simulink model "nonlinear_ss_control_with_reference"  (R2019b)
settings: Solver=ode45  StartTime=0.0  StopTime=700.0  MaxStep=0.001  RelTol=1e-8
settings Model: Creator=Hector  LastModifiedBy=Hector

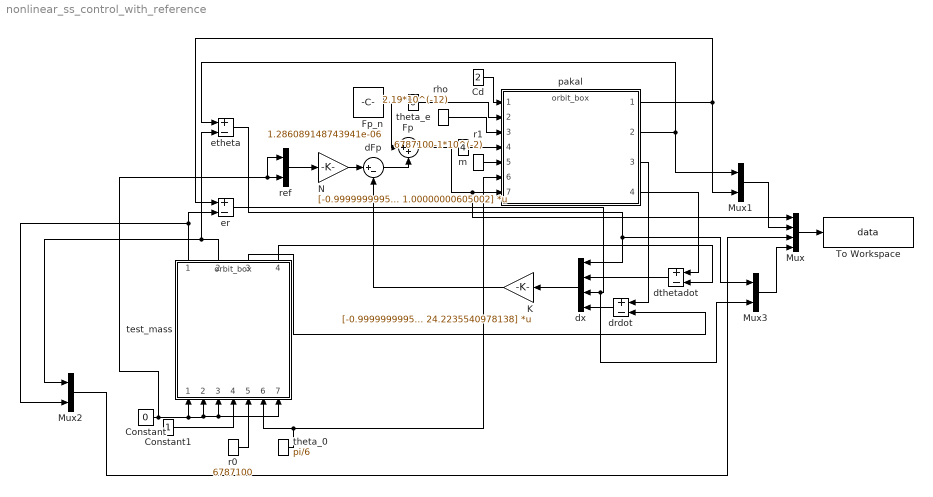
== system nonlinear_ss_control_with_reference ==
  Cd : Constant  Value=2
  Constant : Constant  Value=0
  Constant1 : Constant
  Fp : Sum  Inputs=|++
  Fp_n : Constant  Value=1.286089148743941e-06
  K : Gain  Gain=[-0.999999999517925 4489802.13130477 1.00112038113525 24.2235540978138]  Multiplication=Matrix(K*u)
  Mux : Mux
  Mux1 : Mux  Inputs=2
  Mux2 : Mux  Inputs=2
  Mux3 : Mux  Inputs=2
  N : Gain  Gain=[-0.999999999517925 1.00000000605002]  Multiplication=Matrix(K*u)
  To Workspace : ToWorkspace  VariableName=data  SaveFormat=Timeseries  SampleTime=-1
  dFp : Sum  Inputs=|+-
  drdot : Sum  Inputs=+-
  dthetadot : Sum  Inputs=+-
  dx : Mux
  er : Sum  Inputs=+-
  etheta : Sum  Inputs=+-
  m : Constant  Value=4
  pakal : ModelReference  ModelNameDialog=orbit_box.slx  SimulationMode=Normal  ModelReferenceVersion=1.38
  r0 : Constant  Value=6787100
  r1 : Constant  Value=6787100-1*10^(-2)
  ref : Mux  Inputs=2
  rho : Constant  Value=2.19*10^(-12)
  test_mass : ModelReference  ModelNameDialog=orbit_box.slx  SimulationMode=Normal  ModelReferenceVersion=1.38
  theta_0 : Constant  Value=pi/6
  theta_e : Constant  Value=0
  wires:
  pakal/1 -> Mux1/2, er/1
  er/1 -> Mux3/2, dx/3
  dFp/1 -> Fp/2
  etheta/1 -> Mux3/1, dx/1
  Fp_n/1 -> Fp/1
  r0/1 -> test_mass/5
  ref/1 -> N/1
  Constant1/1 -> test_mass/4
  theta_0/1 -> pakal/6, test_mass/6
  N/1 -> dFp/1
  K/1 -> dFp/2
  pakal/2 -> Mux1/1, etheta/1
  Fp/1 -> Mux/1, pakal/7
  dx/1 -> K/1
  pakal/3 -> drdot/1
  r1/1 -> pakal/5
  m/1 -> pakal/4
  rho/1 -> pakal/3
  theta_e/1 -> pakal/2
  Cd/1 -> pakal/1
  dthetadot/1 -> dx/2
  pakal/4 -> dthetadot/1
  test_mass/4 -> dthetadot/2
  drdot/1 -> dx/4
  test_mass/3 -> drdot/2
  Mux/1 -> To Workspace/1
  test_mass/1 -> Mux2/2, er/2
  test_mass/2 -> Mux2/1, etheta/2
  Mux1/1 -> Mux/2
  Mux2/1 -> Mux/3
  Constant/1 -> ref/1, ref/2, test_mass/1, test_mass/7, test_mass/3, test_mass/2
  Mux3/1 -> Mux/4
